simulink model "StateSwitch"  (Simulink 8.0)
settings: Solver=FixedStepDiscrete  StartTime=0.0  StopTime=5  FixedStep=Ts  RelTol=1e-3
undefined symbols (not defined in the file): DiscIntNeverNeededParam, Ts
libraries: simulink x2
settings Model: Creator=LukePH  LastModifiedBy=Luke
settings OptimizationCC: ExpressionDepthLimit=128
settings DebuggingCC: StateNameClashWarn=none
settings CodeAppCC: CustomSymbolStrType=$N$R$M_T  InternalIdentifier=Shortened

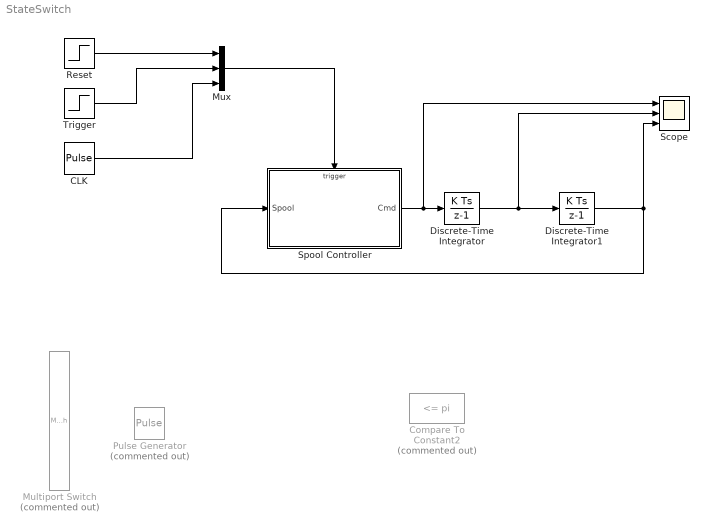
== system StateSwitch ==
  CLK : DiscretePulseGenerator  PulseType=Time based  Period=2*Ts  PulseWidth=50
  Compare To Constant2 : simulink/Logic and Bit Operations/Compare To Constant  Commented=on  relop=<=  const=pi  OutDataTypeStr=uint8
  Discrete-Time Integrator : DiscreteIntegrator  SampleTime=Ts  ICPrevOutput=DiscIntNeverNeededParam  ICPrevScaledInput=DiscIntNeverNeededParam
  Discrete-Time Integrator1 : DiscreteIntegrator  SampleTime=Ts  ICPrevOutput=DiscIntNeverNeededParam  ICPrevScaledInput=DiscIntNeverNeededParam
  Multiport Switch : MultiPortSwitch  Commented=on
  Mux : Mux  Inputs=3
  Pulse Generator : DiscretePulseGenerator  Commented=on  PulseType=Time based  Period=10  PulseWidth=5
  Reset : Step  Time=.1  Before=1  After=0  SampleTime=0
  Scope : Scope  NumInputPorts=3
      settings: YMin=-5~-5~-5  YMax=5~5~5
  Spool Controller : Stateflow chart  RequirementInfo="{}  %GIDa_33442fbe_5776_46ae_820c_e485a662037e"  TreatAsAtomicUnit=on
  Trigger : Step  Time=.5  SampleTime=0
  wires:
  Trigger/1 -> Mux/2
  Mux/1 -> Spool Controller/Trigger
  Spool Controller/1(Cmd) -> Scope/1, Discrete-Time Integrator/1
  Discrete-Time Integrator/1 -> Scope/2, Discrete-Time Integrator1/1
  Discrete-Time Integrator1/1 -> Spool Controller/1(Spool), Scope/3
  Reset/1 -> Mux/1
  CLK/1 -> Mux/3

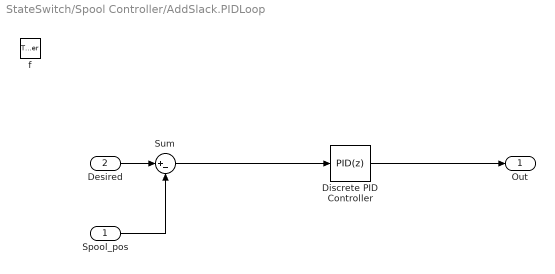
== system StateSwitch/Spool Controller/AddSlack.PIDLoop ==
  Spool_pos : Inport
  Desired : Inport  Port=2
  f : TriggerPort  TriggerType=function-call
      settings: CopyFcn=Stateflow.SLINSF.SimulinkMan.removeBlockPreDeleteFcn  PreDeleteFcn=Stateflow.SLINSF.SimulinkMan.unsafePredeleteFcn
  Discrete PID Controller : simulink/Continuous/PID Controller  Controller=PID  TimeDomain=Discrete-time  SampleTime=-1  IntegratorMethod=Forward Euler  FilterMethod=Forward Euler  Form=Parallel  P=1  I=1  D=0  N=100  InitialConditionSource=internal  InitialConditionForIntegrator=0  InitialConditionForFilter=0  ExternalReset=none  LimitOutput=off  UpperSaturationLimit=inf  LowerSaturationLimit=-inf  LinearizeAsGain=off  AntiWindupMode=none  Kb=1  TrackingMode=off  Kt=1  PParamMin=[]  PParamMax=[]  IParamMin=[]  IParamMax=[]  DParamMin=[]  DParamMax=[]  NParamMin=[]  NParamMax=[]  KbParamMin=[]  KbParamMax=[]  KtParamMin=[]  KtParamMax=[]  POutMin=[]  POutMax=[]  IOutMin=[]  IOutMax=[]  DOutMin=[]  DOutMax=[]  NOutMin=[]  NOutMax=[]  KbOutMin=[]  KbOutMax=[]  KtOutMin=[]  KtOutMax=[]  IntegratorOutMin=[]  IntegratorOutMax=[]  FilterOutMin=[]  FilterOutMax=[]  SumOutMin=[]  SumOutMax=[]  SumI1OutMin=[]  SumI1OutMax=[]  SumI2OutMin=[]  SumI2OutMax=[]  SumI3OutMin=[]  SumI3OutMax=[]  SumDOutMin=[]  SumDOutMax=[]  SaturationOutMin=[]  SaturationOutMax=[]  IntegratorContinuousStateAttributes=''  IntegratorStateMustResolveToSignalObject=off  IntegratorRTWStateStorageClass=Auto  FilterContinuousStateAttributes=''  FilterStateMustResolveToSignalObject=off  FilterRTWStateStorageClass=Auto
  Sum : Sum  Inputs=|+-
  Out : Outport
  wires:
  Spool_pos/1 -> Sum/2
  Desired/1 -> Sum/1
  Sum/1 -> Discrete PID Controller/1
  Discrete PID Controller/1 -> Out/1

== stateflow chart Spool Controller ==
  state AddSlack
    entry: Cmd = 0;
    during: Cmd = PIDLoop(Spool, 3);
    state Out = PIDLoop(Spool_pos,Desired) [function]
  state PassiveSpool
    entry: Cmd = 0;
  state HoldTight
    entry: Cmd  = 6;
  (default) -> PassiveSpool
  HoldTight -> AddSlack : Trig
  AddSlack -> PassiveSpool : [Spool >=3]
  PassiveSpool -> HoldTight : Reset
  data: Out function_output double; Spool_pos function_input double; Desired function_input double; Spool input double; Cmd output double
  events: Reset input FALLING_EDGE_EVENT; Trig input RISING_EDGE_EVENT; CLK input EITHER_EDGE_EVENT
